simulink model "alt_turn"  (R2019b)
settings: Solver=VariableStepAuto  StartTime=0.0  StopTime=250  RelTol=1e-3
values from neighbouring files (symbols this model uses):
  A_alh = [[A_long; [sin(theta0) -cos(theta0) 0 u0*cos(theta0)]] [0;0;0;0;0]]    [Project.m]
  A_lat = [Yv/m Yp/m (Yr/m)-u0 g*cos(theta0); I_xx*Lv+I_xz*Nv I_xx*Lp+I_xz*Np I_xx*Lr+I_xz*Nr 0; I_zz*Nv+I_xz*Lv I_zz*Np+I_xz*Lp I_zz*Nr+I_xz*Lr 0; 0 1 tan(theta0) 0]    [Project.m]
  B_alh = [B_long; [0 0]]    [Project.m]
  B_lat = [Yda/m Ydr/m; I_xx*Lda+I_xz*Nda I_xx*Ldr+I_xz*Ndr; I_zz*Nda+I_xz*Lda I_zz*Ndr+I_xz*Ldr; 0 0]    [Project.m]
  g = 32.2    [CRJ330Config.m]    (also in Data.mat)
  u0 = 726.5928    [CRJ330Config.m]    (also in Data.mat)
libraries: simulink x3
settings Model: Creator=BALKRISHNA SHAH  LastModifiedBy=BALKRISHNA SHAH

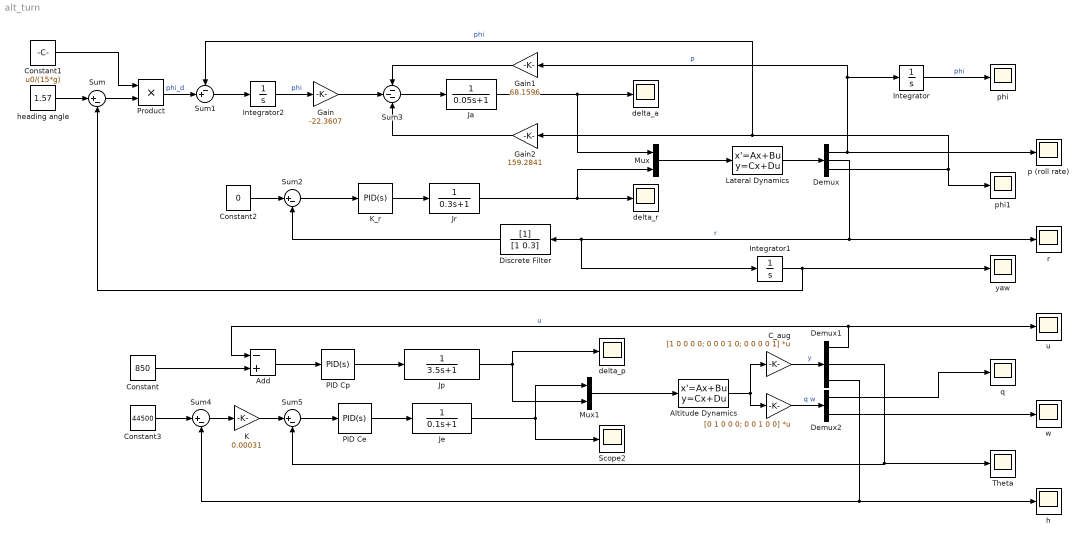
== system alt_turn ==
  " " : Gain  Gain=[0 1 0 0 0; 0 0 1 0 0]  Multiplication=Matrix(K*u)
  Add : Sum  Inputs=-+
  Altitude Dynamics : StateSpace  A=A_alh  B=B_alh  C=eye(5)  D=zeros(5,2)  InitialCondition=[800;0;0;0;41500]
  C_aug : Gain  Gain=[1 0 0 0 0; 0 0 0 1 0; 0 0 0 0 1]  Multiplication=Matrix(K*u)
  Constant : Constant  Value=850
  Constant1 : Constant  Value=u0/(15*g)
  Constant2 : Constant  Value=0
  Constant3 : Constant  Value=44500
  Demux : Demux  Outputs=3
  Demux1 : Demux  Outputs=3
  Demux2 : Demux  Outputs=2
  Discrete Filter : DiscreteFilter  Denominator=[1 0.3]
  Gain : Gain  Gain=-22.3607
  Gain1 : Gain  Gain=68.1596
  Gain2 : Gain  Gain=159.2841
  Integrator : Integrator
  Integrator1 : Integrator
  Integrator2 : Integrator
  "Ja " : TransferFcn  Denominator=[0.05 1]
  Je : TransferFcn  Denominator=[0.1 1]
  Jp : TransferFcn  Denominator=[3.5 1]
  Jr : TransferFcn  Denominator=[0.3 1]
  K : Gain  Gain=0.00031
  K_r : simulink/Continuous/PID Controller  Controller=PID  Form=Parallel  TimeDomain=Continuous-time  SampleTime=-1  IntegratorMethod=Forward Euler  FilterMethod=Forward Euler  ControllerParametersSource=internal  P=0.257  I=0.0578  D=0.5798  UseFilter=on  N=0.7895  TunerSelectOption=Transfer Function Based (PID Tuner App)  InitialConditionSource=internal  InitialConditionForIntegrator=0  InitialConditionForFilter=0  DifferentiatorICPrevScaledInput=0  ExternalReset=none  TrackingMode=off  Kt=1  LimitOutput=off  UpperSaturationLimit=inf  LowerSaturationLimit=-inf  LinearizeAsGain=on  AntiWindupMode=none  Kb=1  POutMin=[]  POutMax=[]  IOutMin=[]  IOutMax=[]  DOutMin=[]  DOutMax=[]  NOutMin=[]  NOutMax=[]  SumOutMin=[]  SumOutMax=[]  SaturationOutMin=[]  SaturationOutMax=[]  PParamMin=[]  PParamMax=[]  IParamMin=[]  IParamMax=[]  DParamMin=[]  DParamMax=[]  NParamMin=[]  NParamMax=[]  KbParamMin=[]  KbParamMax=[]  KtParamMin=[]  KtParamMax=[]  KbOutMin=[]  KbOutMax=[]  KtOutMin=[]  KtOutMax=[]  IntegratorOutMin=[]  IntegratorOutMax=[]  FilterOutMin=[]  FilterOutMax=[]  SumI1OutMin=[]  SumI1OutMax=[]  SumI2OutMin=[]  SumI2OutMax=[]  SumI3OutMin=[]  SumI3OutMax=[]  SumI4OutMin=[]  SumI4OutMax=[]  SumDOutMin=[]  SumDOutMax=[]  DifferentiatorOutMin=[]  DifferentiatorOutMax=[]  FilterDiffOutCoefMin=[]  FilterDiffOutCoefMax=[]  ReciprocalOutMin=[]  ReciprocalOutMax=[]  SumDenOutMin=[]  SumDenOutMax=[]  SumNumOutMin=[]  SumNumOutMax=[]  DivideOutMin=[]  DivideOutMax=[]  IntegratorContinuousStateAttributes=''  IntegratorStateMustResolveToSignalObject=off  IntegratorRTWStateStorageClass=Auto  FilterContinuousStateAttributes=''  FilterStateMustResolveToSignalObject=off  FilterRTWStateStorageClass=Auto  ParallelPVariant=InternalParameters  IdealPVariant=Disabled  IVariant=InternalParameters  DVariant=InternalParameters  IntegratorVariant=Continuous  SatVariant=Disabled  AWVariant=Passthrough  PCopyVariant=Disabled  TRVariant=Disabled  FdbkBlocksVariant=Forward  IdealPFdbkVariant=Disabled  SatFdbkVariant=Disabled  DerivativeFilterVariant=ContFilter  NVariant=InternalParameters  NCopyVariant=Disabled  FilterICVariant=InternalICsFilter  IntegratorICVariant=InternalICs  ExternalResetVariant=Disabled  TRSumVariant=Passthrough  SumFdbkVariant=Disabled  SumVariant=Sum_PID
  Lateral Dynamics : StateSpace  A=A_lat  B=B_lat  C=[0 1 0 0; 0 0 1 0; 0 0 0 1]  D=zeros(3,2)  InitialCondition=[0;0;0;0]
  Mux : Mux  Inputs=2
  Mux1 : Mux  Inputs=2
  PID Ce : simulink/Continuous/PID Controller  Controller=PID  Form=Parallel  TimeDomain=Continuous-time  SampleTime=-1  IntegratorMethod=Forward Euler  FilterMethod=Forward Euler  ControllerParametersSource=internal  P=7.1*(-0.0083661)*10  I=-0.0083661  D=3.5^2*(-0.0083661)  UseFilter=on  N=100  TunerSelectOption=Transfer Function Based (PID Tuner App)  InitialConditionSource=internal  InitialConditionForIntegrator=0  InitialConditionForFilter=0  DifferentiatorICPrevScaledInput=0  ExternalReset=none  TrackingMode=off  Kt=1  LimitOutput=off  UpperSaturationLimit=inf  LowerSaturationLimit=-inf  LinearizeAsGain=on  AntiWindupMode=none  Kb=1  POutMin=[]  POutMax=[]  IOutMin=[]  IOutMax=[]  DOutMin=[]  DOutMax=[]  NOutMin=[]  NOutMax=[]  SumOutMin=[]  SumOutMax=[]  SaturationOutMin=[]  SaturationOutMax=[]  PParamMin=[]  PParamMax=[]  IParamMin=[]  IParamMax=[]  DParamMin=[]  DParamMax=[]  NParamMin=[]  NParamMax=[]  KbParamMin=[]  KbParamMax=[]  KtParamMin=[]  KtParamMax=[]  KbOutMin=[]  KbOutMax=[]  KtOutMin=[]  KtOutMax=[]  IntegratorOutMin=[]  IntegratorOutMax=[]  FilterOutMin=[]  FilterOutMax=[]  SumI1OutMin=[]  SumI1OutMax=[]  SumI2OutMin=[]  SumI2OutMax=[]  SumI3OutMin=[]  SumI3OutMax=[]  SumI4OutMin=[]  SumI4OutMax=[]  SumDOutMin=[]  SumDOutMax=[]  DifferentiatorOutMin=[]  DifferentiatorOutMax=[]  FilterDiffOutCoefMin=[]  FilterDiffOutCoefMax=[]  ReciprocalOutMin=[]  ReciprocalOutMax=[]  SumDenOutMin=[]  SumDenOutMax=[]  SumNumOutMin=[]  SumNumOutMax=[]  DivideOutMin=[]  DivideOutMax=[]  IntegratorContinuousStateAttributes=''  IntegratorStateMustResolveToSignalObject=off  IntegratorRTWStateStorageClass=Auto  FilterContinuousStateAttributes=''  FilterStateMustResolveToSignalObject=off  FilterRTWStateStorageClass=Auto  ParallelPVariant=InternalParameters  IdealPVariant=Disabled  IVariant=InternalParameters  DVariant=InternalParameters  IntegratorVariant=Continuous  SatVariant=Disabled  AWVariant=Passthrough  PCopyVariant=Disabled  TRVariant=Disabled  FdbkBlocksVariant=Forward  IdealPFdbkVariant=Disabled  SatFdbkVariant=Disabled  DerivativeFilterVariant=ContFilter  NVariant=InternalParameters  NCopyVariant=Disabled  FilterICVariant=InternalICsFilter  IntegratorICVariant=InternalICs  ExternalResetVariant=Disabled  TRSumVariant=Passthrough  SumFdbkVariant=Disabled  SumVariant=Sum_PID
  PID Cp : simulink/Continuous/PID Controller  Controller=PID  Form=Parallel  TimeDomain=Continuous-time  SampleTime=-1  IntegratorMethod=Forward Euler  FilterMethod=Forward Euler  ControllerParametersSource=internal  P=7.4*0.038971  I=0.038971  D=3.7^2*0.038971  UseFilter=on  N=100  TunerSelectOption=Transfer Function Based (PID Tuner App)  InitialConditionSource=internal  InitialConditionForIntegrator=0  InitialConditionForFilter=0  DifferentiatorICPrevScaledInput=0  ExternalReset=none  TrackingMode=off  Kt=1  LimitOutput=off  UpperSaturationLimit=inf  LowerSaturationLimit=-inf  LinearizeAsGain=on  AntiWindupMode=none  Kb=1  POutMin=[]  POutMax=[]  IOutMin=[]  IOutMax=[]  DOutMin=[]  DOutMax=[]  NOutMin=[]  NOutMax=[]  SumOutMin=[]  SumOutMax=[]  SaturationOutMin=[]  SaturationOutMax=[]  PParamMin=[]  PParamMax=[]  IParamMin=[]  IParamMax=[]  DParamMin=[]  DParamMax=[]  NParamMin=[]  NParamMax=[]  KbParamMin=[]  KbParamMax=[]  KtParamMin=[]  KtParamMax=[]  KbOutMin=[]  KbOutMax=[]  KtOutMin=[]  KtOutMax=[]  IntegratorOutMin=[]  IntegratorOutMax=[]  FilterOutMin=[]  FilterOutMax=[]  SumI1OutMin=[]  SumI1OutMax=[]  SumI2OutMin=[]  SumI2OutMax=[]  SumI3OutMin=[]  SumI3OutMax=[]  SumI4OutMin=[]  SumI4OutMax=[]  SumDOutMin=[]  SumDOutMax=[]  DifferentiatorOutMin=[]  DifferentiatorOutMax=[]  FilterDiffOutCoefMin=[]  FilterDiffOutCoefMax=[]  ReciprocalOutMin=[]  ReciprocalOutMax=[]  SumDenOutMin=[]  SumDenOutMax=[]  SumNumOutMin=[]  SumNumOutMax=[]  DivideOutMin=[]  DivideOutMax=[]  IntegratorContinuousStateAttributes=''  IntegratorStateMustResolveToSignalObject=off  IntegratorRTWStateStorageClass=Auto  FilterContinuousStateAttributes=''  FilterStateMustResolveToSignalObject=off  FilterRTWStateStorageClass=Auto  ParallelPVariant=InternalParameters  IdealPVariant=Disabled  IVariant=InternalParameters  DVariant=InternalParameters  IntegratorVariant=Continuous  SatVariant=Disabled  AWVariant=Passthrough  PCopyVariant=Disabled  TRVariant=Disabled  FdbkBlocksVariant=Forward  IdealPFdbkVariant=Disabled  SatFdbkVariant=Disabled  DerivativeFilterVariant=ContFilter  NVariant=InternalParameters  NCopyVariant=Disabled  FilterICVariant=InternalICsFilter  IntegratorICVariant=InternalICs  ExternalResetVariant=Disabled  TRSumVariant=Passthrough  SumFdbkVariant=Disabled  SumVariant=Sum_PID
  Product : Product
  Scope2 : Scope
  Sum{,2,4..5} (4 alike) : Sum  Inputs=|+-
  Sum1 : Sum  Inputs=-+|
  Sum3 : Sum  Inputs=---
  Theta : Scope
  delta_a : Scope
  delta_p : Scope
  "delta_r " : Scope
  h : Scope
  "heading angle " : Constant  Value=1.57
  p (roll rate) : Scope
  phi : Scope
  phi1 : Scope
  q : Scope
  r : Scope
  u : Scope
  w : Scope
  yaw : Scope
  wires:
  "heading angle "/1 -> Sum/1
  Sum/1 -> Product/2
  Constant1/1 -> Product/1
  Product/1 -> Sum1/2  "phi_d"
  Sum1/1 -> Integrator2/1
  "Ja "/1 -> delta_a/1, Mux/1
  Lateral Dynamics/1 -> Demux/1
  Jr/1 -> Mux/2, "delta_r "/1
  Demux/1 -> p (roll rate)/1, Gain1/1, Integrator/1  "p"
  Integrator/1 -> phi/1  "phi"
  Sum2/1 -> K_r/1
  Constant2/1 -> Sum2/1
  Gain/1 -> Sum3/2
  Sum3/1 -> "Ja "/1
  Demux/2 -> r/1, Integrator1/1, Discrete Filter/1  "r"
  Integrator1/1 -> yaw/1, Sum/2
  K_r/1 -> Jr/1
  Discrete Filter/1 -> Sum2/2
  Demux/3 -> phi1/1, Sum1/1, Gain2/1  "phi"
  Integrator2/1 -> Gain/1  "phi"
  Gain1/1 -> Sum3/1
  Gain2/1 -> Sum3/3
  Constant/1 -> Add/2
  Sum5/1 -> PID Ce/1
  Demux2/1 -> q/1
  PID Ce/1 -> Je/1
  Jp/1 -> Mux1/2, delta_p/1
  Je/1 -> Scope2/1, Mux1/1
  " "/1 -> Demux2/1  "q w"
  Constant3/1 -> Sum4/1
  K/1 -> Sum5/1
  Demux2/2 -> w/1
  Demux1/2 -> Sum5/2, Theta/1
  Altitude Dynamics/1 -> " "/1, C_aug/1
  Demux1/3 -> Sum4/2, h/1
  Sum4/1 -> K/1
  Add/1 -> PID Cp/1
  C_aug/1 -> Demux1/1  "y"
  Demux1/1 -> Add/1, u/1  "u"
  Mux/1 -> Lateral Dynamics/1
  Mux1/1 -> Altitude Dynamics/1
  PID Cp/1 -> Jp/1
